simulink model "tqdtqr_rebuild_V3"  (R2021b)
settings: Solver=VariableStepAuto  StartTime=0.0  StopTime=10.0  RelTol=1e-3
undefined symbols (not defined in the file): ATQD_AfterTqMinGain_X_Deg, ATQD_APSCreepBaseTqD_X_kph, ATQD_APSCreepBaseTqD_Y_Deg, ATQD_APSCreepBaseTqR_X_kph, ATQD_APSCreepBaseTqR_Y_Deg, ATQD_APSCreepIterm_X_kph, ATQD_APSCreepIterm_Y_kph, ATQD_APSCreepPterm_X_kph, ATQD_APSCreepPterm_Y_kph, ATQD_APSDecReq_X_kph, ATQD_APSDecReq_Y_mps2, ATQD_APSDecReqCMD_X_kph, ATQD_APSDecReqTs_X_pct, ATQD_APSDecTimeGain_X_Deg, ATQD_APSDecTimeGain_Y_s, ATQD_APSReqLowSpd_X_Deg, ATQD_AutoHoldReleaseBPS_X_Deg, ATQD_AWDLoadTrqnsGain_X_kg, ATQD_AWDLoadTrqnsGain_Y_pct, ATQD_BOSEnBPSPosn_X_kph, ATQD_BOSMap_X_rpm, ATQD_BOSMap_Y_pct, ATQD_CreepBaseTqD_X_kph, ATQD_CreepBaseTqD_Y_Deg, ATQD_CreepBaseTqR_X_kph, ATQD_CreepBaseTqR_Y_Deg, ATQD_CreepBPSDisPosn_X_Deg, ATQD_CreepBPSDisPosnR_X_Deg, ATQD_CreepBPSEnPosn_X_Deg, ATQD_CreepBPSEnPosnR_X_Deg, ATQD_CreepDeltaTq_X_kph, ATQD_CreepIterm_X_kph, ATQD_CreepIterm_Y_kph, ATQD_CreepItermMaxLimit_X_pct, ATQD_CreepPreloadTime_X_kph, ATQD_CreepPreloadTq_X_kph, ATQD_CreepPreloadTq_Y_s, ATQD_CreepProtTq_X_Deg, ATQD_CreepPterm_X_kph, ATQD_CreepPterm_Y_kph, ATQD_CreepRrTqSpRat_X_rpm, ATQD_CreepRrTqSpRat_Y_Nm, ATQD_CreepTargetSpdD_X_pct, ATQD_CreepTargetSpdR_X_pct, ATQD_CreepUpLimitTq_X_rpm, ATQD_DecIneOPDHoldEnDelay_X_Deg, ATQD_DecIneOPDHoldEnDelay_Y_bar, ATQD_ECOTqMapD_X_rpm, ATQD_ECOTqMapD_Y_pct, ATQD_EMTqMapD_X_rpm, ATQD_EMTqMapD_Y_pct, ATQD_EOPDTqMapDCon_X_rpm, ATQD_EOPDTqMapDCon_Y_Deg, ATQD_EstInitVehWeight_X_c, ATQD_FAfterTqCMDGain_X_rpm, ATQD_FAfterTqCMDGain_Y_pct, ATQD_ForceLowSpd_X_Deg, ATQD_ForcePLimitSpd_X_Deg, ATQD_FrLossMAPLowV_X_rpm, ATQD_FrLossMAPLowV_Y_Nm ... (+949)
libraries: simulink x235, hcu_lib x208, tqr x63, tqd x6
(part 21 of 37)

== system tqdtqr_rebuild_V3/Input_Convert/Main function/Front//Rear zero point transfer/Negative Rate limit Determination ==
  VTQD_TqTargetShaftSpd_rpm : Inport
  VTQR_FEDUWhlTqReqSmoothDelay_Nm : Inport  Port=2
  VTQR_EVDriveMode_enum : Inport  Port=3
  Constant1 : Constant  Value=ENUM_DRIVEMODE_ECO
  Constant2 : Constant  Value=ENUM_DRIVEMODE_NRM
  Constant3 : Constant  Value=ENUM_DRIVEMODE_SPORT
  Constant7 : Constant  Value=ENUM_DRIVEMODE_ECO
  Constant8 : Constant  Value=ENUM_DRIVEMODE_NRM
  Constant9 : Constant  Value=ENUM_DRIVEMODE_SPORT
  Equal{1..3,5..6,8} (6 alike) : RelationalOperator  Operator===  OutDataTypeStr=boolean  RndMeth=Simplest
  If1 : If  NumInputs=3  IfExpression=u1~= 0  ElseIfExpressions=u2 ~= 0, u3 ~= 0  ShowElse=off
  If2 : If  NumInputs=3  IfExpression=u1~= 0  ElseIfExpressions=u2 ~= 0, u3 ~= 0  ShowElse=off
  Merge1 : Merge  Inputs=3
  Merge2 : Merge  Inputs=3
  Mux : Mux  Inputs=2
  VTQR_FrNegRateLimitDecE_Nm : Subsystem  TreatAsAtomicUnit=on
  VTQR_FrNegRateLimitDecN_Nm : Subsystem  TreatAsAtomicUnit=on
  VTQR_FrNegRateLimitDecS_Nm : Subsystem  TreatAsAtomicUnit=on
  VTQR_FrNegRateLimitIncE_Nm : Subsystem  TreatAsAtomicUnit=on
  VTQR_FrNegRateLimitIncN_Nm : Subsystem  TreatAsAtomicUnit=on
  VTQR_FrNegRateLimitIncS_Nm : Subsystem  TreatAsAtomicUnit=on
  VTQR_NegRateLimit_mux : Outport
  wires:
  VTQR_EVDriveMode_enum/1 -> [VTQR_EVDriveMode_enum]
  VTQR_FEDUWhlTqReqSmoothDelay_Nm/1 -> [VTQR_FEDUWhlTqReqSmoothDelay_Nm]
  VTQD_TqTargetShaftSpd_rpm/1 -> [VTQD_TqTargetShaftSpd_rpm]
  Mux/1 -> VTQR_NegRateLimit_mux/1  "VTQR_NegRateLimit_mux"
  Merge1/1 -> Mux/1  "VTQR_NegRateLimitInc_Nm"
  Constant7/1 -> Equal5/2
  Constant9/1 -> Equal8/2
  Constant8/1 -> Equal6/2
  [VTQR_EVDriveMode_enum] -> Equal5/1
  [VTQR_EVDriveMode_enum] -> Equal8/1
  [VTQR_EVDriveMode_enum] -> Equal6/1
  Equal6/1 -> If1/1
  Equal5/1 -> If1/2
  Equal8/1 -> If1/3
  [VTQD_TqTargetShaftSpd_rpm] -> VTQR_FrNegRateLimitIncN_Nm/1(VTQD_TqTargetShaftSpd_rpm)
  [VTQR_FEDUWhlTqReqSmoothDelay_Nm] -> VTQR_FrNegRateLimitIncN_Nm/2(VTQR_FEDUWhlTqReqSmoothDelay_Nm)
  If1/1 -> VTQR_FrNegRateLimitIncN_Nm/Action
  VTQR_FrNegRateLimitIncN_Nm/1(VTQR_FrNegRateLimitIncN_Nm) -> Merge1/1
  [VTQD_TqTargetShaftSpd_rpm] -> VTQR_FrNegRateLimitIncE_Nm/1(VTQD_TqTargetShaftSpd_rpm)
  [VTQR_FEDUWhlTqReqSmoothDelay_Nm] -> VTQR_FrNegRateLimitIncE_Nm/2(VTQR_FEDUWhlTqReqSmoothDelay_Nm)
  [VTQR_FEDUWhlTqReqSmoothDelay_Nm] -> VTQR_FrNegRateLimitIncS_Nm/2(VTQR_FEDUWhlTqReqSmoothDelay_Nm)
  [VTQD_TqTargetShaftSpd_rpm] -> VTQR_FrNegRateLimitIncS_Nm/1(VTQD_TqTargetShaftSpd_rpm)
  If1/3 -> VTQR_FrNegRateLimitIncS_Nm/Action
  If1/2 -> VTQR_FrNegRateLimitIncE_Nm/Action
  VTQR_FrNegRateLimitIncS_Nm/1(VTQR_FrNegRateLimitIncS_Nm) -> Merge1/3
  VTQR_FrNegRateLimitIncE_Nm/1(VTQR_FrNegRateLimitIncE_Nm) -> Merge1/2
  VTQR_FrNegRateLimitDecN_Nm/1(VTQR_FrNegRateLimitDecN_Nm) -> Merge2/1
  If2/3 -> VTQR_FrNegRateLimitDecS_Nm/Action
  Equal1/1 -> If2/2
  VTQR_FrNegRateLimitDecS_Nm/1(VTQR_FrNegRateLimitDecS_Nm) -> Merge2/3
  [VTQD_TqTargetShaftSpd_rpm] -> VTQR_FrNegRateLimitDecS_Nm/1(VTQD_TqTargetShaftSpd_rpm)
  [VTQR_FEDUWhlTqReqSmoothDelay_Nm] -> VTQR_FrNegRateLimitDecS_Nm/2(VTQR_FEDUWhlTqReqSmoothDelay_Nm)
  If2/1 -> VTQR_FrNegRateLimitDecN_Nm/Action
  [VTQR_FEDUWhlTqReqSmoothDelay_Nm] -> VTQR_FrNegRateLimitDecE_Nm/2(VTQR_FEDUWhlTqReqSmoothDelay_Nm)
  VTQR_FrNegRateLimitDecE_Nm/1(VTQR_FrNegRateLimitDecE_Nm) -> Merge2/2
  [VTQR_EVDriveMode_enum] -> Equal2/1
  [VTQR_EVDriveMode_enum] -> Equal3/1
  If2/2 -> VTQR_FrNegRateLimitDecE_Nm/Action
  Equal3/1 -> If2/3
  Constant3/1 -> Equal3/2
  Constant2/1 -> Equal2/2
  Equal2/1 -> If2/1
  [VTQR_EVDriveMode_enum] -> Equal1/1
  [VTQD_TqTargetShaftSpd_rpm] -> VTQR_FrNegRateLimitDecN_Nm/1(VTQD_TqTargetShaftSpd_rpm)
  [VTQR_FEDUWhlTqReqSmoothDelay_Nm] -> VTQR_FrNegRateLimitDecN_Nm/2(VTQR_FEDUWhlTqReqSmoothDelay_Nm)
  [VTQD_TqTargetShaftSpd_rpm] -> VTQR_FrNegRateLimitDecE_Nm/1(VTQD_TqTargetShaftSpd_rpm)
  Constant1/1 -> Equal1/2
  Merge2/1 -> Mux/2  "VTQR_NegRateLimitDec_Nm"

== system tqdtqr_rebuild_V3/Input_Convert/Main function/Front//Rear zero point transfer/Negative Rate limit Determination1 ==
  VTQD_TqTargetShaftSpd_rpm : Inport
  VTQR_REDUWhlTqReqSmoothDelay_Nm : Inport  Port=2
  VTQR_EVDriveMode_enum : Inport  Port=3
  Constant1 : Constant  Value=ENUM_DRIVEMODE_ECO
  Constant2 : Constant  Value=ENUM_DRIVEMODE_NRM
  Constant3 : Constant  Value=ENUM_DRIVEMODE_SPORT
  Constant7 : Constant  Value=ENUM_DRIVEMODE_ECO
  Constant8 : Constant  Value=ENUM_DRIVEMODE_NRM
  Constant9 : Constant  Value=ENUM_DRIVEMODE_SPORT
  Equal{1..3,5..6,8} (6 alike) : RelationalOperator  Operator===  OutDataTypeStr=boolean  RndMeth=Simplest
  If1 : If  NumInputs=3  IfExpression=u1~= 0  ElseIfExpressions=u2 ~= 0, u3 ~= 0  ShowElse=off
  If2 : If  NumInputs=3  IfExpression=u1~= 0  ElseIfExpressions=u2 ~= 0, u3 ~= 0  ShowElse=off
  Merge1 : Merge  Inputs=3
  Merge2 : Merge  Inputs=3
  Mux : Mux  Inputs=2
  VTQR_RrNegRateLimitDecE_Nm : Subsystem  TreatAsAtomicUnit=on
  VTQR_RrNegRateLimitDecN_Nm : Subsystem  TreatAsAtomicUnit=on
  VTQR_RrNegRateLimitDecS_Nm : Subsystem  TreatAsAtomicUnit=on
  VTQR_RrNegRateLimitIncE_Nm : Subsystem  TreatAsAtomicUnit=on
  VTQR_RrNegRateLimitIncN_Nm : Subsystem  TreatAsAtomicUnit=on
  VTQR_RrNegRateLimitIncS_Nm : Subsystem  TreatAsAtomicUnit=on
  VTQR_NegRateLimit_mux : Outport
  wires:
  Merge2/1 -> Mux/2  "VTQR_NegRateLimitDec_Nm"
  Constant1/1 -> Equal1/2
  [VTQD_TqTargetShaftSpd_rpm] -> VTQR_RrNegRateLimitDecE_Nm/1(VTQD_TqTargetShaftSpd_rpm)
  [VTQR_REDUWhlTqReqSmoothDelay_Nm] -> VTQR_RrNegRateLimitDecN_Nm/2(VTQR_REDUWhlTqReqSmoothDelay_Nm)
  [VTQD_TqTargetShaftSpd_rpm] -> VTQR_RrNegRateLimitDecN_Nm/1(VTQD_TqTargetShaftSpd_rpm)
  [VTQR_EVDriveMode_enum] -> Equal1/1
  Equal2/1 -> If2/1
  Constant2/1 -> Equal2/2
  Constant3/1 -> Equal3/2
  Equal3/1 -> If2/3
  If2/2 -> VTQR_RrNegRateLimitDecE_Nm/Action
  [VTQR_EVDriveMode_enum] -> Equal3/1
  [VTQR_EVDriveMode_enum] -> Equal2/1
  VTQR_RrNegRateLimitDecE_Nm/1(VTQR_RrNegRateLimitDecE_Nm) -> Merge2/2
  [VTQR_REDUWhlTqReqSmoothDelay_Nm] -> VTQR_RrNegRateLimitDecE_Nm/2(VTQR_REDUWhlTqReqSmoothDelay_Nm)
  If2/1 -> VTQR_RrNegRateLimitDecN_Nm/Action
  [VTQR_REDUWhlTqReqSmoothDelay_Nm] -> VTQR_RrNegRateLimitDecS_Nm/2(VTQR_REDUWhlTqReqSmoothDelay_Nm)
  [VTQD_TqTargetShaftSpd_rpm] -> VTQR_RrNegRateLimitDecS_Nm/1(VTQD_TqTargetShaftSpd_rpm)
  VTQR_RrNegRateLimitDecS_Nm/1(VTQR_RrNegRateLimitDecS_Nm) -> Merge2/3
  Equal1/1 -> If2/2
  If2/3 -> VTQR_RrNegRateLimitDecS_Nm/Action
  VTQR_RrNegRateLimitDecN_Nm/1(VTQR_RrNegRateLimitDecN_Nm) -> Merge2/1
  VTQR_RrNegRateLimitIncE_Nm/1(VTQR_RrNegRateLimitIncE_Nm) -> Merge1/2
  VTQR_RrNegRateLimitIncS_Nm/1(VTQR_RrNegRateLimitIncS_Nm) -> Merge1/3
  If1/2 -> VTQR_RrNegRateLimitIncE_Nm/Action
  If1/3 -> VTQR_RrNegRateLimitIncS_Nm/Action
  [VTQD_TqTargetShaftSpd_rpm] -> VTQR_RrNegRateLimitIncS_Nm/1(VTQD_TqTargetShaftSpd_rpm)
  [VTQR_REDUWhlTqReqSmoothDelay_Nm] -> VTQR_RrNegRateLimitIncS_Nm/2(VTQR_REDUWhlTqReqSmoothDelay_Nm)
  [VTQR_REDUWhlTqReqSmoothDelay_Nm] -> VTQR_RrNegRateLimitIncE_Nm/2(VTQR_REDUWhlTqReqSmoothDelay_Nm)
  [VTQD_TqTargetShaftSpd_rpm] -> VTQR_RrNegRateLimitIncE_Nm/1(VTQD_TqTargetShaftSpd_rpm)
  VTQR_RrNegRateLimitIncN_Nm/1(VTQR_RrNegRateLimitIncN_Nm) -> Merge1/1
  If1/1 -> VTQR_RrNegRateLimitIncN_Nm/Action
  [VTQR_REDUWhlTqReqSmoothDelay_Nm] -> VTQR_RrNegRateLimitIncN_Nm/2(VTQR_REDUWhlTqReqSmoothDelay_Nm)
  [VTQD_TqTargetShaftSpd_rpm] -> VTQR_RrNegRateLimitIncN_Nm/1(VTQD_TqTargetShaftSpd_rpm)
  Equal8/1 -> If1/3
  Equal5/1 -> If1/2
  Equal6/1 -> If1/1
  [VTQR_EVDriveMode_enum] -> Equal6/1
  [VTQR_EVDriveMode_enum] -> Equal8/1
  [VTQR_EVDriveMode_enum] -> Equal5/1
  Constant8/1 -> Equal6/2
  Constant9/1 -> Equal8/2
  Constant7/1 -> Equal5/2
  Merge1/1 -> Mux/1  "VTQR_NegRateLimitInc_Nm"
  Mux/1 -> VTQR_NegRateLimit_mux/1  "VTQR_NegRateLimit_mux"
  VTQD_TqTargetShaftSpd_rpm/1 -> [VTQD_TqTargetShaftSpd_rpm]
  VTQR_REDUWhlTqReqSmoothDelay_Nm/1 -> [VTQR_REDUWhlTqReqSmoothDelay_Nm]
  VTQR_EVDriveMode_enum/1 -> [VTQR_EVDriveMode_enum]

== system tqdtqr_rebuild_V3/Input_Convert/Main function/Front//Rear zero point transfer/Positive Rate limit Determination ==
  VTQD_TqTargetShaftSpd_rpm : Inport
  VTQR_FEDUWhlTqReqSmoothDelay_Nm : Inport  Port=2
  VTQR_EVDriveMode_enum : Inport  Port=3
  Constant1 : Constant  Value=ENUM_DRIVEMODE_ECO
  Constant2 : Constant  Value=ENUM_DRIVEMODE_NRM
  Constant3 : Constant  Value=ENUM_DRIVEMODE_SPORT
  Constant7 : Constant  Value=ENUM_DRIVEMODE_ECO
  Constant8 : Constant  Value=ENUM_DRIVEMODE_NRM
  Constant9 : Constant  Value=ENUM_DRIVEMODE_SPORT
  Equal{1..3,5..6,8} (6 alike) : RelationalOperator  Operator===  OutDataTypeStr=boolean  RndMeth=Simplest
  If1 : If  NumInputs=3  IfExpression=u1~= 0  ElseIfExpressions=u2 ~= 0, u3 ~= 0  ShowElse=off
  If2 : If  NumInputs=3  IfExpression=u1~= 0  ElseIfExpressions=u2 ~= 0, u3 ~= 0  ShowElse=off
  Merge1 : Merge  Inputs=3
  Merge2 : Merge  Inputs=3
  Mux : Mux  Inputs=2
  VTQR_FrPosRateLimitDecE_Nm : Subsystem  TreatAsAtomicUnit=on
  VTQR_FrPosRateLimitDecN_Nm : Subsystem  TreatAsAtomicUnit=on
  VTQR_FrPosRateLimitDecS_Nm : Subsystem  TreatAsAtomicUnit=on
  VTQR_FrPosRateLimitIncE_Nm : Subsystem  TreatAsAtomicUnit=on
  VTQR_FrPosRateLimitIncN_Nm : Subsystem  TreatAsAtomicUnit=on
  VTQR_FrPosRateLimitIncS_Nm : Subsystem  TreatAsAtomicUnit=on
  VTQR_PosRateLimit_mux : Outport
  wires:
  VTQR_EVDriveMode_enum/1 -> [VTQR_EVDriveMode_enum]
  VTQR_FEDUWhlTqReqSmoothDelay_Nm/1 -> [VTQR_FEDUWhlTqReqSmoothDelay_Nm]
  Merge2/1 -> Mux/2  "VTQR_PosRateLimitDec_Nm"
  Constant1/1 -> Equal1/2
  [VTQD_TqTargetShaftSpd_rpm] -> VTQR_FrPosRateLimitDecE_Nm/1(VTQD_TqTargetShaftSpd_rpm)
  [VTQR_FEDUWhlTqReqSmoothDelay_Nm] -> VTQR_FrPosRateLimitDecN_Nm/2(VTQR_FEDUWhlTqReqSmoothDelay_Nm)
  [VTQD_TqTargetShaftSpd_rpm] -> VTQR_FrPosRateLimitDecN_Nm/1(VTQD_TqTargetShaftSpd_rpm)
  [VTQR_EVDriveMode_enum] -> Equal1/1
  Equal2/1 -> If2/1
  Constant2/1 -> Equal2/2
  Constant3/1 -> Equal3/2
  Equal3/1 -> If2/3
  If2/2 -> VTQR_FrPosRateLimitDecE_Nm/Action
  [VTQR_EVDriveMode_enum] -> Equal3/1
  [VTQR_EVDriveMode_enum] -> Equal2/1
  VTQR_FrPosRateLimitDecE_Nm/1(VTQR_FrPosRateLimitDecE_Nm) -> Merge2/2
  [VTQR_FEDUWhlTqReqSmoothDelay_Nm] -> VTQR_FrPosRateLimitDecE_Nm/2(VTQR_FEDUWhlTqReqSmoothDelay_Nm)
  If2/1 -> VTQR_FrPosRateLimitDecN_Nm/Action
  [VTQR_FEDUWhlTqReqSmoothDelay_Nm] -> VTQR_FrPosRateLimitDecS_Nm/2(VTQR_FEDUWhlTqReqSmoothDelay_Nm)
  [VTQD_TqTargetShaftSpd_rpm] -> VTQR_FrPosRateLimitDecS_Nm/1(VTQD_TqTargetShaftSpd_rpm)
  VTQR_FrPosRateLimitDecS_Nm/1(VTQR_FrPosRateLimitDecS_Nm) -> Merge2/3
  Equal1/1 -> If2/2
  If2/3 -> VTQR_FrPosRateLimitDecS_Nm/Action
  VTQR_FrPosRateLimitDecN_Nm/1(VTQR_FrPosRateLimitDecN_Nm) -> Merge2/1
  VTQR_FrPosRateLimitIncE_Nm/1(VTQR_FrPosRateLimitIncE_Nm) -> Merge1/2
  VTQR_FrPosRateLimitIncS_Nm/1(VTQR_FrPosRateLimitIncS_Nm) -> Merge1/3
  If1/2 -> VTQR_FrPosRateLimitIncE_Nm/Action
  If1/3 -> VTQR_FrPosRateLimitIncS_Nm/Action
  [VTQD_TqTargetShaftSpd_rpm] -> VTQR_FrPosRateLimitIncS_Nm/1(VTQD_TqTargetShaftSpd_rpm)
  [VTQR_FEDUWhlTqReqSmoothDelay_Nm] -> VTQR_FrPosRateLimitIncS_Nm/2(VTQR_FEDUWhlTqReqSmoothDelay_Nm)
  [VTQR_FEDUWhlTqReqSmoothDelay_Nm] -> VTQR_FrPosRateLimitIncE_Nm/2(VTQR_FEDUWhlTqReqSmoothDelay_Nm)
  [VTQD_TqTargetShaftSpd_rpm] -> VTQR_FrPosRateLimitIncE_Nm/1(VTQD_TqTargetShaftSpd_rpm)
  VTQR_FrPosRateLimitIncN_Nm/1(VTQR_FrPosRateLimitIncN_Nm) -> Merge1/1
  If1/1 -> VTQR_FrPosRateLimitIncN_Nm/Action
  [VTQR_FEDUWhlTqReqSmoothDelay_Nm] -> VTQR_FrPosRateLimitIncN_Nm/2(VTQR_FEDUWhlTqReqSmoothDelay_Nm)
  [VTQD_TqTargetShaftSpd_rpm] -> VTQR_FrPosRateLimitIncN_Nm/1(VTQD_TqTargetShaftSpd_rpm)
  Equal8/1 -> If1/3
  Equal5/1 -> If1/2
  Equal6/1 -> If1/1
  [VTQR_EVDriveMode_enum] -> Equal6/1
  [VTQR_EVDriveMode_enum] -> Equal8/1
  [VTQR_EVDriveMode_enum] -> Equal5/1
  Constant8/1 -> Equal6/2
  Constant9/1 -> Equal8/2
  Constant7/1 -> Equal5/2
  Merge1/1 -> Mux/1  "VTQR_PosRateLimitInc_Nm"
  Mux/1 -> VTQR_PosRateLimit_mux/1  "VTQR_PosRateLimit_mux"
  VTQD_TqTargetShaftSpd_rpm/1 -> [VTQD_TqTargetShaftSpd_rpm]

== system tqdtqr_rebuild_V3/Input_Convert/Main function/Front//Rear zero point transfer/Positive Rate limit Determination1 ==
  VTQD_TqTargetShaftSpd_rpm : Inport
  VTQR_REDUWhlTqReqSmoothDelay_Nm : Inport  Port=2
  VTQR_EVDriveMode_enum : Inport  Port=3
  Constant1 : Constant  Value=ENUM_DRIVEMODE_ECO
  Constant2 : Constant  Value=ENUM_DRIVEMODE_NRM
  Constant3 : Constant  Value=ENUM_DRIVEMODE_SPORT
  Constant7 : Constant  Value=ENUM_DRIVEMODE_ECO
  Constant8 : Constant  Value=ENUM_DRIVEMODE_NRM
  Constant9 : Constant  Value=ENUM_DRIVEMODE_SPORT
  Equal{1..3,5..6,8} (6 alike) : RelationalOperator  Operator===  OutDataTypeStr=boolean  RndMeth=Simplest
  If1 : If  NumInputs=3  IfExpression=u1~= 0  ElseIfExpressions=u2 ~= 0, u3 ~= 0  ShowElse=off
  If2 : If  NumInputs=3  IfExpression=u1~= 0  ElseIfExpressions=u2 ~= 0, u3 ~= 0  ShowElse=off
  Merge1 : Merge  Inputs=3
  Merge2 : Merge  Inputs=3
  Mux : Mux  Inputs=2
  VTQR_RrPosRateLimitDecE_Nm : Subsystem  TreatAsAtomicUnit=on
  VTQR_RrPosRateLimitDecN_Nm : Subsystem  TreatAsAtomicUnit=on
  VTQR_RrPosRateLimitDecS_Nm : Subsystem  TreatAsAtomicUnit=on
  VTQR_RrPosRateLimitIncE_Nm : Subsystem  TreatAsAtomicUnit=on
  VTQR_RrPosRateLimitIncN_Nm : Subsystem  TreatAsAtomicUnit=on
  VTQR_RrPosRateLimitIncS_Nm : Subsystem  TreatAsAtomicUnit=on
  VTQR_PosRateLimit_mux : Outport
  wires:
  Mux/1 -> VTQR_PosRateLimit_mux/1  "VTQR_PosRateLimit_mux"
  Merge1/1 -> Mux/1  "VTQR_PosRateLimitInc_Nm"
  Constant7/1 -> Equal5/2
  Constant9/1 -> Equal8/2
  Constant8/1 -> Equal6/2
  [VTQR_EVDriveMode_enum] -> Equal5/1
  [VTQR_EVDriveMode_enum] -> Equal8/1
  [VTQR_EVDriveMode_enum] -> Equal6/1
  Equal6/1 -> If1/1
  Equal5/1 -> If1/2
  Equal8/1 -> If1/3
  [VTQD_TqTargetShaftSpd_rpm] -> VTQR_RrPosRateLimitIncN_Nm/1(VTQD_TqTargetShaftSpd_rpm)
  [VTQR_REDUWhlTqReqSmoothDelay_Nm] -> VTQR_RrPosRateLimitIncN_Nm/2(VTQR_REDUWhlTqReqSmoothDelay_Nm)
  If1/1 -> VTQR_RrPosRateLimitIncN_Nm/Action
  VTQR_RrPosRateLimitIncN_Nm/1(VTQR_RrPosRateLimitIncN_Nm) -> Merge1/1
  [VTQD_TqTargetShaftSpd_rpm] -> VTQR_RrPosRateLimitIncE_Nm/1(VTQD_TqTargetShaftSpd_rpm)
  [VTQR_REDUWhlTqReqSmoothDelay_Nm] -> VTQR_RrPosRateLimitIncE_Nm/2(VTQR_REDUWhlTqReqSmoothDelay_Nm)
  [VTQR_REDUWhlTqReqSmoothDelay_Nm] -> VTQR_RrPosRateLimitIncS_Nm/2(VTQR_REDUWhlTqReqSmoothDelay_Nm)
  [VTQD_TqTargetShaftSpd_rpm] -> VTQR_RrPosRateLimitIncS_Nm/1(VTQD_TqTargetShaftSpd_rpm)
  If1/3 -> VTQR_RrPosRateLimitIncS_Nm/Action
  If1/2 -> VTQR_RrPosRateLimitIncE_Nm/Action
  VTQR_RrPosRateLimitIncS_Nm/1(VTQR_RrPosRateLimitIncS_Nm) -> Merge1/3
  VTQR_RrPosRateLimitIncE_Nm/1(VTQR_RrPosRateLimitIncE_Nm) -> Merge1/2
  VTQR_RrPosRateLimitDecN_Nm/1(VTQR_RrPosRateLimitDecN_Nm) -> Merge2/1
  If2/3 -> VTQR_RrPosRateLimitDecS_Nm/Action
  Equal1/1 -> If2/2
  VTQR_RrPosRateLimitDecS_Nm/1(VTQR_RrPosRateLimitDecS_Nm) -> Merge2/3
  [VTQD_TqTargetShaftSpd_rpm] -> VTQR_RrPosRateLimitDecS_Nm/1(VTQD_TqTargetShaftSpd_rpm)
  [VTQR_REDUWhlTqReqSmoothDelay_Nm] -> VTQR_RrPosRateLimitDecS_Nm/2(VTQR_REDUWhlTqReqSmoothDelay_Nm)
  If2/1 -> VTQR_RrPosRateLimitDecN_Nm/Action
  [VTQR_REDUWhlTqReqSmoothDelay_Nm] -> VTQR_RrPosRateLimitDecE_Nm/2(VTQR_REDUWhlTqReqSmoothDelay_Nm)
  VTQR_RrPosRateLimitDecE_Nm/1(VTQR_RrPosRateLimitDecE_Nm) -> Merge2/2
  [VTQR_EVDriveMode_enum] -> Equal2/1
  [VTQR_EVDriveMode_enum] -> Equal3/1
  If2/2 -> VTQR_RrPosRateLimitDecE_Nm/Action
  Equal3/1 -> If2/3
  Constant3/1 -> Equal3/2
  Constant2/1 -> Equal2/2
  Equal2/1 -> If2/1
  [VTQR_EVDriveMode_enum] -> Equal1/1
  [VTQD_TqTargetShaftSpd_rpm] -> VTQR_RrPosRateLimitDecN_Nm/1(VTQD_TqTargetShaftSpd_rpm)
  [VTQR_REDUWhlTqReqSmoothDelay_Nm] -> VTQR_RrPosRateLimitDecN_Nm/2(VTQR_REDUWhlTqReqSmoothDelay_Nm)
  [VTQD_TqTargetShaftSpd_rpm] -> VTQR_RrPosRateLimitDecE_Nm/1(VTQD_TqTargetShaftSpd_rpm)
  Constant1/1 -> Equal1/2
  Merge2/1 -> Mux/2  "VTQR_PosRateLimitDec_Nm"
  VTQD_TqTargetShaftSpd_rpm/1 -> [VTQD_TqTargetShaftSpd_rpm]
  VTQR_REDUWhlTqReqSmoothDelay_Nm/1 -> [VTQR_REDUWhlTqReqSmoothDelay_Nm]
  VTQR_EVDriveMode_enum/1 -> [VTQR_EVDriveMode_enum]

== system tqdtqr_rebuild_V3/Input_Convert/Main function/Tq distribution function/AWD_Ratio ==
  VVMC_APSActive_flg : Inport
  VTQD_CreepPrLoadEnable_flg : Inport  Port=2
  VTQD_RrRatioWithRrSR_rat : Inport  Port=3
  VTQD_CreepEnable_flg : Inport  Port=4
  VTQD_OrigRrDriverRatio_rat : Inport  Port=5
  VTQD_CreepRrTqSpRat_rat : Inport  Port=6
  VTQD_RrTqSRRateTs_c : Inport  Port=7
  task_time_s : Inport  Port=8
  Action Port : ActionPort  ActionPortLabel=elseif(u2 ~= 0)
  AND : Logic  AllPortsSameDT=off  OutDataTypeStr=boolean
  AND2 : Logic  AllPortsSameDT=off  OutDataTypeStr=boolean
  Constant : Constant  Value=ONE_FLOAT
  Constant10 : Constant  Value=KTQD_AWDRrRatio_rat_ovrdflg  VectorParams1D=off  SampleTime=-1
  Constant11 : Constant  Value=KTQD_AWDRrRatio_rat_ovrdval  VectorParams1D=off  SampleTime=-1
  Constant12 : Constant  Value=KTQD_DrvSelPwrTrainSW_flg  VectorParams1D=off  SampleTime=-1
  Constant14 : Constant  Value=KTQD_CreepWhlRatioSW_flg
  Constant17 : Constant  Value=KTQD_AWDTqRatioSW_enum
  Constant18 : Constant  Value=KTQD_DriverSelPowerTrain_enum
  Constant19 : Constant  OutDataTypeStr=uint8
  Constant20 : Constant  Value=KTQD_AWDTqRatioSW_enum
  Constant21 : Constant  Value=2  OutDataTypeStr=uint8
  Constant3 : Constant  Value=ENUM_DRIVETRAIN_FWD  VectorParams1D=off  SampleTime=-1
  Constant4 : Constant  Value=ENUM_DRIVETRAIN_AWD  VectorParams1D=off  SampleTime=-1
  Constant6 : Constant  Value=KTQD_AWDFWDSelRRatio_rat  VectorParams1D=off  SampleTime=-1
  Constant7 : Constant  Value=KTQD_AWDRWDSelRRatio_rat  VectorParams1D=off  SampleTime=-1
  Constant8 : Constant  Value=KTQD_AWDFrRatio_rat_ovrdflg  VectorParams1D=off  SampleTime=-1
  Constant9 : Constant  Value=KTQD_AWDFrRatio_rat_ovrdval  VectorParams1D=off  SampleTime=-1
  Equal1 : RelationalOperator  Operator=~=  OutDataTypeStr=boolean  RndMeth=Simplest
  Equal3 : RelationalOperator  Operator===  OutDataTypeStr=boolean  RndMeth=Simplest
  Equal6 : RelationalOperator  Operator===  OutDataTypeStr=boolean  RndMeth=Simplest
  Equal7 : RelationalOperator  Operator===  OutDataTypeStr=boolean  RndMeth=Simplest
  FirstOrderFilter : hcu_lib/Basic_Blocks/FirstOrderFilter
  LiuzgSwitch2 : Switch  Criteria=u2 ~= 0
      settings: AttributesFormatString=<%<Criteria>>
  LiuzgSwitch4 : Switch  Criteria=u2 ~= 0
      settings: AttributesFormatString=<%<Criteria>>
  LiuzgSwitch5 : Switch  Criteria=u2 ~= 0
      settings: AttributesFormatString=<%<Criteria>>
  OR : Logic  Operator=OR  AllPortsSameDT=off  OutDataTypeStr=boolean
  OR1 : Logic  AllPortsSameDT=off  OutDataTypeStr=boolean
  OR3 : Logic  Operator=OR  AllPortsSameDT=off  OutDataTypeStr=boolean
  Saturation : Saturate  UpperLimit=KTQD_RrEDUTqDistrictMax_gain  LowerLimit=KTQD_RrEDUTqDistrictMin_gain
      settings: AttributesFormatString=|
      | <%<UpperLimit>>
      | <%<LowerLimit>>
  Subtract : Sum  Inputs=+-
  Switch : Switch  Criteria=u2 > Threshold
  Switch1 : Switch  Criteria=u2 > Threshold
  Switch3 : Switch  Criteria=u2 > Threshold
  VTQD_FrRatio_AWD : Outport
  VTQD_RrRatio_AWD : Outport  Port=2
  wires:
  [VTQD_RrTqSRRateTs_c] -> FirstOrderFilter/3
  [task_time_s] -> FirstOrderFilter/2
  FirstOrderFilter/1 -> LiuzgSwitch4/3
  LiuzgSwitch2/1 -> FirstOrderFilter/1
  task_time_s/1 -> [task_time_s]
  VTQD_RrTqSRRateTs_c/1 -> [VTQD_RrTqSRRateTs_c]
  [VTQD_CreepRrTqSpRat_rat] -> LiuzgSwitch2/1
  VTQD_CreepRrTqSpRat_rat/1 -> [VTQD_CreepRrTqSpRat_rat]
  VTQD_OrigRrDriverRatio_rat/1 -> [VTQD_OrigRrDriverRatio_rat]
  OR3/1 -> Switch3/2
  Equal7/1 -> OR3/2
  Constant20/1 -> Equal7/1
  Constant21/1 -> Equal7/2
  AND2/1 -> OR3/1
  [VTQD_CreepEnable_flg] -> AND2/2
  Equal6/1 -> AND2/1
  Constant19/1 -> Equal6/2
  Constant17/1 -> Equal6/1
  [VTQD_RrRatioWithRrSR_rat] -> Switch3/1
  [VTQD_OrigRrDriverRatio_rat] -> Switch3/3
  Switch3/1 -> LiuzgSwitch2/3  "VTQD_FitRrDriverRatio_rat"
  Constant6/1 -> LiuzgSwitch5/1
  Constant7/1 -> LiuzgSwitch5/3
  VTQD_RrRatioWithRrSR_rat/1 -> [VTQD_RrRatioWithRrSR_rat]
  VTQD_CreepEnable_flg/1 -> [VTQD_CreepEnable_flg]
  Constant14/1 -> OR1/2
  OR1/1 -> LiuzgSwitch2/2
  AND/1 -> LiuzgSwitch4/2
  Equal1/1 -> AND/1
  Constant12/1 -> AND/2
  Constant10/1 -> Switch1/2
  Constant11/1 -> Switch1/1
  Constant9/1 -> Switch/1
  Constant8/1 -> Switch/2
  Switch1/1 -> VTQD_RrRatio_AWD/1
  Switch/1 -> VTQD_FrRatio_AWD/1
  Subtract/1 -> Switch/3
  Constant18/1 -> [VINP_DriverSelPowerTrain_enum]  "VINP_DriverSelPowerTrain_enum"
  LiuzgSwitch4/1 -> Saturation/1
  Equal3/1 -> LiuzgSwitch5/2
  [VINP_DriverSelPowerTrain_enum] -> Equal3/1
  Constant3/1 -> Equal3/2
  LiuzgSwitch5/1 -> LiuzgSwitch4/1
  Constant4/1 -> Equal1/2
  [VINP_DriverSelPowerTrain_enum] -> Equal1/1
  VTQD_CreepPrLoadEnable_flg/1 -> [VTQD_CreepPrLoadEnable_flg]
  VVMC_APSActive_flg/1 -> [VVMC_APSActive_flg]
  [VVMC_APSActive_flg] -> OR/1
  [VTQD_CreepPrLoadEnable_flg] -> OR/2
  OR/1 -> OR1/1
  Saturation/1 -> Subtract/2, Switch1/3
  Constant/1 -> Subtract/1

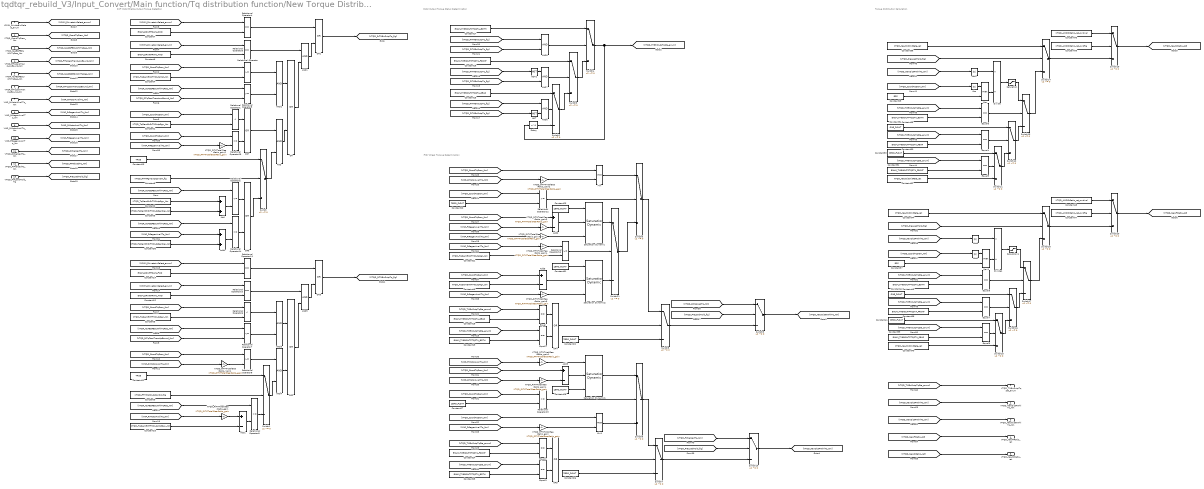
== system tqdtqr_rebuild_V3/Input_Convert/Main function/Tq distribution function/New Torque Distribution ==
  note: Rr/Fr Motor Enable Output Torque Detection
  note: Motor Output Torque Status Determination
  note: Fr/Rr Wheel Torqrue Determination
  note: Torque Distribution Calculation
  VPMM_DrivetrainSelect_enum : Inport
  VTQD_CoordTqDem_Nm : Inport  Port=2
  VTQR_NoABSFEDUWhlTqReq_Nm : Inport  Port=3
  VTQR_FrTqZeroTransLowBound_Nm : Inport  Port=4
  VTQR_NoABSREDUWhlTqReq_Nm : Inport  Port=5
  VTQR_RrTqZeroTransUpBound_Nm : Inport  Port=6
  VINP_RrMotorAvailTq_Nm : Inport  Port=7
  VINP_RrRegenAvailTq_Nm : Inport  Port=8
  VINP_FrMotorAvailTq_Nm : Inport  Port=9
  VINP_FrRegenAvailTq_Nm : Inport  Port=10
  VTQD_RrPreloadTq_Nm : Inport  Port=11
  VTQD_FrPreloadTq_Nm : Inport  Port=12
  VTQD_PreLoadHold_flg : Inport  Port=13
  AND{,1..8} (9 alike) : Logic  AllPortsSameDT=off  OutDataTypeStr=boolean
  Abs{,1..3} (4 alike) : Abs
  Add : Sum
  Add{1..3,5} (4 alike) : Sum  Inputs=+-
  Add4 : Sum
  Constant{1..2,21,49} (4 alike) : Constant  Value=KTQD_TqDemEnRrTMOutpRgn_Nm
  Constant10 : Constant  Value=KTQD_TqDemEnFrTMOutpMotDev_Nm
  Constant11 : Constant  Value=TRUE
  Constant12 : Constant  Value=ENUM_DRIVETRAIN_AWD
  Constant13 : Constant  Value=TRUE
  Constant14 : Constant  Value=ENUM_DRIVETRAIN_FWD
  Constant{15,18,30,39} (4 alike) : Constant  Value=ENUM_TMENOUTPTQSTA_REAR
  Constant{16,24,31,38} (4 alike) : Constant  Value=ENUM_TMENOUTPTQSTA_FRONT
  Constant{17,19,25,35,43} (5 alike) : Constant  Value=ENUM_TMENOUTPTQSTA_BOTH
  Constant{20,22..23,26..28,33,41,51} (9 alike) : Constant  Value=ZERO_FLOAT
  Constant29 : Constant  Value=EPS
  Constant3 : Constant  Value=KTQD_TqDemEnRrTMOutpRgnDev_Nm
  Constant{32,36,40,44} (4 alike) : Constant  Value=KTQD_NewDistInitRate_rat
  Constant34 : Constant  Value=ONE_FLOAT
  Constant37 : Constant  Value=EPS
  Constant4 : Constant  Value=KTQD_TqDemEnRrTMOutpMot_Nm
  Constant42 : Constant  Value=ONE_FLOAT
  Constant45 : Constant  Value=KTQD_AWDRrRatio_rat_ovrdflg
  Constant46 : Constant  Value=KTQD_AWDRrRatio_rat_ovrdval
  Constant47 : Constant  Value=KTQD_AWDRrRatio_rat_ovrdflg
  Constant48 : Constant  Value=KTQD_AWDRrRatio_rat_ovrdval
  Constant5 : Constant  Value=KTQD_TqDemEnFrTMOutpRgn_Nm
  Constant50 : Constant  Value=KTQD_TqDemEnRrTMOutpRgnDev_Nm
  Constant6 : Constant  Value=ENUM_DRIVETRAIN_AWD
  Constant7 : Constant  Value=ENUM_DRIVETRAIN_RWD
  Constant8 : Constant  Value=KTQD_RrTMRgnOutpConSW_flg
  Constant9 : Constant  Value=KTQD_FrTMMotOutpConSW_flg
  Delay : Delay  DelayLength=1  InitialCondition=uint8(0)
      settings: AttributesFormatString=%<InitialCondition>
  Divide : Product  Inputs=*/
  Divide1 : Product  Inputs=*/
  Equal{,1..9} (10 alike) : RelationalOperator  Operator===  OutDataTypeStr=boolean  RndMeth=Simplest
  KTQD_FrTMTotalGearRatio_gain{,1..4} (5 alike) : Gain  Gain=KTQD_FrTMTotalGearRatio_gain
  KTQD_RrTMTotalGearRatio_gain{,1..5} (6 alike) : Gain  Gain=KTQD_RrTMTotalGearRatio_gain
  Max : MinMax  Function=max  Inputs=2
  Max1 : MinMax  Function=max  Inputs=2
  Min : MinMax  Inputs=2
  Min1 : MinMax  Function=max  Inputs=2
  NOT : Logic  Operator=NOT  AllPortsSameDT=off  OutDataTypeStr=boolean
  NOT2 : Logic  Operator=NOT  AllPortsSameDT=off  OutDataTypeStr=boolean
  OR{,1..7} (8 alike) : Logic  Operator=OR  AllPortsSameDT=off  OutDataTypeStr=boolean
  Relational Operator{,5,8..9,12..13,16} (7 alike) : RelationalOperator  OutDataTypeStr=boolean  RndMeth=Simplest
  Relational Operator1 : RelationalOperator  Operator=<  OutDataTypeStr=boolean  RndMeth=Simplest
  Relational Operator{3..4,10..11} (4 alike) : RelationalOperator  Operator===  OutDataTypeStr=boolean  RndMeth=Simplest
  Relational Operator{2,7,14..15} (4 alike) : RelationalOperator  Operator=<=  OutDataTypeStr=boolean  RndMeth=Simplest
  Relational Operator6 : RelationalOperator  Operator=<  OutDataTypeStr=boolean  RndMeth=Simplest
  Saturation : Saturate  UpperLimit=single(1)  LowerLimit=single(0)
      settings: AttributesFormatString=|
      | UpperLimit:%<UpperLimit>
      | LowerLimi:%<LowerLimit>
  Saturation Dynamic : simulink/Discontinuities/Saturation Dynamic  OutMin=[]  OutMax=[]  OutDataTypeStr=Inherit: Same as second input  OutDataType=fixdt(1, 16)  OutScaling=2^-10  DoSatur=off
  Saturation Dynamic1 : simulink/Discontinuities/Saturation Dynamic  OutMin=[]  OutMax=[]  OutDataTypeStr=Inherit: Same as second input  OutDataType=fixdt(1, 16)  OutScaling=2^-10  DoSatur=off
  Saturation Dynamic2 : simulink/Discontinuities/Saturation Dynamic  OutMin=[]  OutMax=[]  OutDataTypeStr=Inherit: Same as second input  OutDataType=fixdt(1, 16)  OutScaling=2^-10  DoSatur=off
  Saturation1 : Saturate  UpperLimit=single(1)  LowerLimit=single(0)
      settings: AttributesFormatString=|
      | UpperLimit:%<UpperLimit>
      | LowerLimi:%<LowerLimit>
  Switch{,1..21} (22 alike) : Switch  Criteria=u2 ~= 0
      settings: AttributesFormatString=%<Criteria>
  VTQD_TMEnOutpTqSta_enum : Outport
  VTQD_NewDistFrWhlTq_Nm : Outport  Port=2
  VTQD_NewDistRrWhlTq_Nm : Outport  Port=3
  VTQD_NewFrRatio_rat : Outport  Port=4
  VTQD_NewRrRatio_rat : Outport  Port=5
  wires:
  VTQD_CoordTqDem_Nm/1 -> [VTQD_CoordTqDem_Nm]
  [VTQD_TMEnOutpTqSta_enum] -> VTQD_TMEnOutpTqSta_enum/1
  Constant21/1 -> Relational Operator16/2
  [VTQD_NewDistRrWhlTq_Nm] -> VTQD_NewDistRrWhlTq_Nm/1
  Relational Operator1/1 -> OR7/1
  VTQD_RrPreloadTq_Nm/1 -> [VTQD_RrPreloadTq_Nm]
  [VTQD_NewDistFrWhlTq_Nm] -> VTQD_NewDistFrWhlTq_Nm/1
  VTQR_NoABSFEDUWhlTqReq_Nm/1 -> [VTQR_NoABSFEDUWhlTqReq_Nm]
  Switch19/1 -> [VTQD_NewRrRatio_rat]  "VTQD_NewRrRatio_rat"
  Relational Operator14/1 -> OR6/2
  OR7/1 -> AND/1
  Add4/1 -> Relational Operator14/2
  Constant50/1 -> Add4/2
  VINP_RrRegenAvailTq_Nm/1 -> [VINP_RrRegenAvailTq_Nm]
  VTQD_PreLoadHold_flg/1 -> [VTQD_PreLoadHold_flg]
  Switch21/1 -> Switch6/3
  Saturation Dynamic/1 -> Switch21/1
  KTQD_FrTMTotalGearRatio_gain3/1 -> Add2/2
  [VTQD_CoordTqDem_Nm] -> Relational Operator15/1
  Switch13/1 -> Switch14/3
  Constant47/1 -> Switch20/2
  Constant49/1 -> Add5/2
  [VINP_RrRegenAvailTq_Nm] -> KTQD_RrTMTotalGearRatio_gain5/1
  [VTQD_PreLoadHold_flg] -> Switch14/2
  Equal6/1 -> Switch13/2
  Constant15/1 -> Switch2/1
  [VTQD_NewRrRatio_rat] -> VTQD_NewRrRatio_rat/1
  Add5/1 -> Saturation Dynamic2/2
  Saturation/1 -> Switch13/1
  [VINP_FrRegenAvailTq_Nm] -> KTQD_FrTMTotalGearRatio_gain/1
  [VINP_FrRegenAvailTq_Nm] -> KTQD_FrTMTotalGearRatio_gain3/1
  Constant24/1 -> Equal2/2
  Constant33/1 -> Switch11/1
  Constant23/1 -> Saturation Dynamic/1
  Constant30/1 -> Equal4/2
  [VTQD_NewDistRrWhlTq_Nm] -> Abs1/1
  Saturation Dynamic1/1 -> Switch8/1
  Constant22/1 -> Switch5/3
  KTQD_RrTMTotalGearRatio_gain1/1 -> Relational Operator8/2
  [VINP_FrRegenAvailTq_Nm] -> Add4/1
  Relational Operator10/1 -> AND5/1
  Constant32/1 -> Switch11/3
  Abs1/1 -> Divide/1
  Switch1/1 -> AND4/2
  Divide/1 -> Saturation/1
  Constant19/1 -> Equal1/2
  [VTQD_FrTMEnOutpTq_flg] -> AND7/2
  KTQD_FrTMTotalGearRatio_gain1/1 -> Saturation Dynamic1/1
  Constant29/1 -> Max/2
  KTQD_RrTMTotalGearRatio_gain3/1 -> Saturation Dynamic/3
  Max/1 -> Divide/2
  Constant27/1 -> Relational Operator13/2
  [VTQD_RrPreloadTq_Nm] -> Switch9/1
  [VTQD_CoordTqDem_Nm] -> Abs/1
  Constant46/1 -> Switch19/1
  Constant16/1 -> Switch3/1
  Constant5/1 -> Relational Operator6/2
  KTQD_FrTMTotalGearRatio_gain2/1 -> Relational Operator15/2
  [VINP_RrRegenAvailTq_Nm] -> KTQD_RrTMTotalGearRatio_gain3/1
  Switch8/1 -> Switch7/1
  Add3/1 -> Saturation Dynamic1/2
  [VPMM_DrivetrainSelect_enum] -> Relational Operator3/1
  Switch5/1 -> Switch9/3
  Switch7/1 -> Switch10/3
  Switch9/1 -> [VTQD_NewDistRrWhlTq_Nm]  "VTQD_NewDistRrWhlTq_Nm"
  Relational Operator13/1 -> Switch8/2
  [VTQR_NoABSFEDUWhlTqReq_Nm] -> Relational Operator14/1
  KTQD_FrTMTotalGearRatio_gain/1 -> Min1/2
  [VINP_FrMotorAvailTq_Nm] -> KTQD_FrTMTotalGearRatio_gain1/1
  [VTQD_CoordTqDem_Nm] -> Relational Operator8/1
  KTQD_RrTMTotalGearRatio_gain4/1 -> Add3/2
  Constant26/1 -> Switch7/3
  Min1/1 -> Switch8/3
  KTQD_FrTMTotalGearRatio_gain4/1 -> Relational Operator16/1
  Relational Operator4/1 -> OR1/1
  VTQR_FrTqZeroTransLowBound_Nm/1 -> [VTQR_FrTqZeroTransLowBound_Nm]
  VINP_FrMotorAvailTq_Nm/1 -> [VINP_FrMotorAvailTq_Nm]
  [VINP_RrMotorAvailTq_Nm] -> KTQD_RrTMTotalGearRatio_gain4/1
  Equal2/1 -> OR5/1
  Constant3/1 -> Add/2
  [VPMM_DrivetrainSelect_enum] -> Relational Operator11/1
  Min/1 -> Switch6/1
  Switch4/1 -> [VTQD_TMEnOutpTqSta_enum], Delay/1  "VTQD_TMEnOutpTqSta_enum"
  Constant35/1 -> Equal6/2
  Constant51/1 -> Saturation Dynamic2/1
  Switch6/1 -> Switch5/1
  KTQD_RrTMTotalGearRatio_gain2/1 -> Min/2
  [VTQD_CoordTqDem_Nm] -> Min/1
  [VTQD_TMEnOutpTqSta_enum] -> Equal6/1
  Relational Operator12/1 -> Switch6/2
  KTQD_RrTMTotalGearRatio_gain/1 -> Add1/1
  Constant25/1 -> Equal3/2
  Add2/1 -> Saturation Dynamic/2
  [VTQD_CoordTqDem_Nm] -> Relational Operator12/1
  [VINP_RrMotorAvailTq_Nm] -> KTQD_RrTMTotalGearRatio_gain2/1
  AND8/1 -> Switch4/2
  [VTQD_TMEnOutpTqSta_enum] -> Equal1/1
  OR4/1 -> Switch5/2
  Relational Operator11/1 -> OR3/1
  Constant20/1 -> Relational Operator12/2
  Switch3/1 -> Switch4/3
  Constant36/1 -> Switch14/1
  [VTQD_CoordTqDem_Nm] -> Relational Operator6/1
  [VTQD_FrTMEnOutpTq_flg] -> NOT/1
  OR5/1 -> Switch7/2
  Add1/1 -> Relational Operator9/2
  Constant9/1 -> Switch1/2
  [VTQD_CoordTqDem_Nm] -> Add2/1
  AND7/1 -> Switch3/2
  Constant18/1 -> Equal/2
  [VTQD_TMEnOutpTqSta_enum] -> Equal3/1
  Relational Operator2/1 -> OR6/1
  AND2/1 -> OR/1
  OR/1 -> AND1/2
  [VTQD_TMEnOutpTqSta_enum] -> Equal/1
  Equal5/1 -> Switch11/2
  [VTQD_RrTMEnOutpTq_flg] -> AND8/1
  [VTQD_RrTMEnOutpTq_flg] -> AND6/1
  VTQR_RrTqZeroTransUpBound_Nm/1 -> [VTQR_RrTqZeroTransUpBound_Nm]
  Constant17/1 -> Switch4/1
  NOT2/1 -> AND7/1
  Relational Operator15/1 -> OR7/2
  [VTQD_RrTMEnOutpTq_flg] -> NOT2/1
  Switch2/1 -> Switch3/3
  Constant11/1 -> Switch1/1
  [VTQD_TMEnOutpTqSta_enum] -> Equal2/1
  Relational Operator9/1 -> Switch1/3
  [VINP_RrMotorAvailTq_Nm] -> KTQD_RrTMTotalGearRatio_gain/1
  Relational Operator8/1 -> AND4/1
  AND5/1 -> OR3/2
  [VTQD_FrTMEnOutpTq_flg] -> AND8/2
  [VTQR_NoABSREDUWhlTqReq_Nm] -> Relational Operator9/1
  OR1/1 -> [VTQD_RrTMEnOutpTq_flg]  "VTQD_RrTMEnOutpTq_flg"
  [VTQR_NoABSREDUWhlTqReq_Nm] -> Relational Operator7/1
  [VPMM_DrivetrainSelect_enum] -> Relational Operator4/1
  AND/1 -> OR/2
  Relational Operator/1 -> AND2/1
  [VTQR_FrTqZeroTransLowBound_Nm] -> Relational Operator5/2
  Constant7/1 -> Relational Operator4/2
  AND1/1 -> OR1/2
  Equal/1 -> OR4/1
  Equal4/1 -> Switch12/2
  [VTQR_NoABSFEDUWhlTqReq_Nm] -> Relational Operator5/1
  [VPMM_DrivetrainSelect_enum] -> Relational Operator10/1
  [VTQD_TMEnOutpTqSta_enum] -> Equal4/1
  Constant45/1 -> Switch19/2
  Relational Operator7/1 -> AND3/2
  Delay/1 -> Switch2/3
  Add/1 -> Relational Operator2/2
  Switch14/1 -> Switch19/3  "VTQD_InitNewRrRatio_rat"
  VTQR_NoABSREDUWhlTqReq_Nm/1 -> [VTQR_NoABSREDUWhlTqReq_Nm]
  [VTQD_CoordTqDem_Nm] -> Relational Operator13/1
  Switch20/1 -> [VTQD_NewFrRatio_rat]  "VTQD_NewFrRatio_rat"
  Constant37/1 -> Max1/2
  Relational Operator5/1 -> AND2/2
  Constant6/1 -> Relational Operator3/2
  [VTQD_CoordTqDem_Nm] -> Abs2/1
  [VTQD_NewDistFrWhlTq_Nm] -> Abs3/1
  Constant13/1 -> Switch/1
  AND6/1 -> Switch2/2
  [VTQD_TMEnOutpTqSta_enum] -> Equal7/1
  Switch12/1 -> Switch13/3
  Switch/1 -> AND/2
  [VTQD_CoordTqDem_Nm] -> Relational Operator/1
  [VTQD_PreLoadHold_flg] -> Switch9/2
  [VINP_FrRegenAvailTq_Nm] -> KTQD_FrTMTotalGearRatio_gain2/1
  [VTQD_TMEnOutpTqSta_enum] -> Equal8/1
  Switch18/1 -> Switch20/3  "VTQD_InitNewFrRatio_rat"
  Divide1/1 -> Saturation1/1
  [VTQR_RrTqZeroTransUpBound_Nm] -> Relational Operator7/2
  [VTQD_CoordTqDem_Nm] -> Min1/1
  Abs3/1 -> Divide1/1
  [VTQD_TMEnOutpTqSta_enum] -> Equal5/1
  [VINP_FrRegenAvailTq_Nm] -> KTQD_FrTMTotalGearRatio_gain4/1
  Equal7/1 -> Switch16/2
  Max1/1 -> Divide1/2
  [VINP_RrMotorAvailTq_Nm] -> KTQD_RrTMTotalGearRatio_gain1/1
  Abs2/1 -> Max1/1
  Relational Operator3/1 -> AND1/1
  VINP_RrMotorAvailTq_Nm/1 -> [VINP_RrMotorAvailTq_Nm]
  Constant28/1 -> Saturation Dynamic1/3
  VINP_FrRegenAvailTq_Nm/1 -> [VINP_FrRegenAvailTq_Nm]
  [VTQD_TMEnOutpTqSta_enum] -> Equal9/1
  Switch15/1 -> Switch16/3
  KTQD_RrTMTotalGearRatio_gain5/1 -> Saturation Dynamic2/3
  VPMM_DrivetrainSelect_enum/1 -> [VPMM_DrivetrainSelect_enum]
  Switch16/1 -> Switch17/3
  [VTQD_CoordTqDem_Nm] -> Relational Operator1/1
  Constant43/1 -> Equal9/2
  OR3/1 -> [VTQD_FrTMEnOutpTq_flg]  "VTQD_FrTMEnOutpTq_flg"
  Constant2/1 -> Add/1
  [VTQR_NoABSFEDUWhlTqReq_Nm] -> Relational Operator2/1
  Switch11/1 -> Switch12/3
  Saturation1/1 -> Switch17/1
  OR6/1 -> Switch/3
  OR2/1 -> AND5/2
  Equal1/1 -> OR4/2
  Constant39/1 -> Equal8/2
  Constant48/1 -> Switch20/1
  Constant44/1 -> Switch18/1
  AND4/1 -> OR2/2
  Constant4/1 -> Relational Operator/2
  Constant31/1 -> Equal5/2
  [VTQD_NewFrRatio_rat] -> VTQD_NewFrRatio_rat/1
  [VTQD_PreLoadHold_flg] -> Switch18/2
  Constant40/1 -> Switch15/3
  Constant1/1 -> Relational Operator1/2
  Constant8/1 -> Switch/2
  [VTQD_FrPreloadTq_Nm] -> Switch10/1
  Relational Operator6/1 -> AND3/1
  Equal3/1 -> OR5/2
  Equal8/1 -> Switch15/2
  Switch10/1 -> [VTQD_NewDistFrWhlTq_Nm]  "VTQD_NewDistFrWhlTq_Nm"
  AND3/1 -> OR2/1
  Constant34/1 -> Switch12/1
  Switch17/1 -> Switch18/3
  Abs/1 -> Max/1
  Constant10/1 -> Add1/2
  Constant38/1 -> Equal7/2
  Constant41/1 -> Switch15/1
  Constant12/1 -> Relational Operator10/2
  Relational Operator16/1 -> Switch21/2
  Constant42/1 -> Switch16/1
  VTQD_FrPreloadTq_Nm/1 -> [VTQD_FrPreloadTq_Nm]
  NOT/1 -> AND6/2
  Constant14/1 -> Relational Operator11/2
  [VTQD_PreLoadHold_flg] -> Switch10/2
  Equal9/1 -> Switch17/2
  [VTQD_CoordTqDem_Nm] -> Add3/1
  Saturation Dynamic2/1 -> Switch21/3
  [VTQD_CoordTqDem_Nm] -> Add5/1

== system tqdtqr_rebuild_V3/Input_Convert/Signal function/OPD Hold/Deceleration Calculation ==
  VTQD_VehActSpd_kph : Inport
  VVMC_LongAcc_Gps : Inport  Port=2
  VTQD_APSReqTimer_s : Inport  Port=3
  VVMC_EstSlope_Deg : Inport  Port=4
  VTQD_APSDecReqA_flg : Inport  Port=5
  VTQD_AutiHoldRelease_flg : Inport  Port=6
  task_time_s : Inport  Port=7
  VTQD_ActAPSPosn_pct : Inport  Port=8
  VTQD_LowIdleAccPedal_flg : Inport  Port=9
  VTQD_OPDHoldForceEn_flg : Inport  Port=10
  AND1 : Logic  Inputs=3  AllPortsSameDT=off  OutDataTypeStr=boolean
  AND4 : Logic  Inputs=3  AllPortsSameDT=off  OutDataTypeStr=boolean
  Add : Sum  Inputs=+-
  Constant1 : Constant  Value=KTQD_APSDecReqMaxTime_s
  Constant13 : Constant  Value=ZERO_FLOAT
  Constant19 : Constant  Value=KTQD_OPDHoldBrkSW_flg
  Constant2 : Constant  Value=KTQD_OPDHoldBrkSW_flg
  Constant21 : Constant  Value=KTQD_OPDHoldDevUpLim_mps2
  Constant22 : Constant  Value=KTQD_OPDHoldDevLowLim_mps2
  Constant43 : Constant  Value=KTQD_APSDecReqMaxSW_flg
  Constant8 : Constant  Value=KVMC_GravityValue_mps2
  Delay : Delay  DelayLength=1
  FirstOrderFilter1 : tqr/TQR/Determine Torque Request/TorqueArbitrament/TorqueSmooth/FirstOrderFilter
  MTQD_APSDecReg_Z_mps2 : Lookup_n-D  BreakpointsForDimension1=ATQD_APSDecReq_Y_mps2  BreakpointsForDimension2=ATQD_APSDecReq_X_kph  Table=MTQD_APSDecReq_Z_mps2  InternalRulePriority=Speed  RndMeth=Simplest  InputSameDT=on
      settings: InputPortMap=u0,u1
  MTQD_APSDecReqCMD_Y_mps2 : Lookup_n-D  NumberOfTableDimensions=1  BreakpointsForDimension1=ATQD_APSDecReqCMD_X_kph  Table=MTQD_APSDecReqCMD_Y_mps2  InternalRulePriority=Speed  RndMeth=Simplest  InputSameDT=on
  MTQD_APSDecReqTs_Y_c : Lookup_n-D  NumberOfTableDimensions=1  BreakpointsForDimension1=ATQD_APSDecReqTs_X_pct  Table=MTQD_APSDecReqTs_Y_c  InternalRulePriority=Speed  RndMeth=Simplest  InputSameDT=on
  MTQD_APSDecTimeGain_Z_c : Lookup_n-D  BreakpointsForDimension1=ATQD_APSDecTimeGain_Y_s  BreakpointsForDimension2=ATQD_APSDecTimeGain_X_Deg  Table=MTQD_APSDecTimeGain_Z_c  InternalRulePriority=Speed  RndMeth=Simplest  InputSameDT=on
      settings: InputPortMap=u0,u1
  MTQD_ForceAPSDecReq_Z_mps2 : Lookup_n-D  BreakpointsForDimension1=ATQD_APSDecReq_Y_mps2  BreakpointsForDimension2=ATQD_APSDecReq_X_kph  Table=MTQD_ForceAPSDecReq_Z_mps2  InternalRulePriority=Speed  RndMeth=Simplest  InputSameDT=on
      settings: InputPortMap=u0,u1
  MTQD_ForceAPSDecTimeGain_Z_c : Lookup_n-D  BreakpointsForDimension1=ATQD_APSDecTimeGain_Y_s  BreakpointsForDimension2=ATQD_APSDecTimeGain_X_Deg  Table=MTQD_ForceAPSDecTimeGain_Z_c  InternalRulePriority=Speed  RndMeth=Simplest  InputSameDT=on
      settings: InputPortMap=u0,u1
  MTQD_PedPressDecTimeGain_Z_c : Lookup_n-D  BreakpointsForDimension1=ATQD_APSDecTimeGain_Y_s  BreakpointsForDimension2=ATQD_APSDecTimeGain_X_Deg  Table=MTQD_PedPressDecTimeGain_Z_c  InternalRulePriority=Speed  RndMeth=Simplest  InputSameDT=on
      settings: InputPortMap=u0,u1
  Max : MinMax  Function=max  Inputs=2
  NOT{1..3,5} (4 alike) : Logic  Operator=NOT  AllPortsSameDT=off  OutDataTypeStr=boolean
  OR : Logic  Operator=OR  AllPortsSameDT=off  OutDataTypeStr=boolean
  Product{,1..4} (5 alike) : Product
  Relational Operator : RelationalOperator  OutDataTypeStr=boolean  RndMeth=Simplest
  SR_Latch : hcu_lib/Basic_Blocks/SR_Latch
  Saturation Dynamic : simulink/Discontinuities/Saturation Dynamic  OutMin=[]  OutMax=[]  OutDataTypeStr=Inherit: Same as second input  OutDataType=fixdt(1, 16)  OutScaling=2^-10  DoSatur=off
  Switch{,1..4,9} (6 alike) : Switch  Criteria=u2 ~= 0
      settings: AttributesFormatString=%<Criteria>
  VTQD_APSDecReq_mps2 : Outport
  wires:
  [VTQD_APSDecReqTs_c] -> FirstOrderFilter1/3
  [VTQD_ActAPSPosn_pct] -> MTQD_APSDecReqTs_Y_c/1
  MTQD_APSDecReqTs_Y_c/1 -> [VTQD_APSDecReqTs_c]  "VTQD_APSDecReqTs_c"
  VTQD_ActAPSPosn_pct/1 -> [VTQD_ActAPSPosn_pct]
  task_time_s/1 -> [task_time_s]
  [task_time_s] -> FirstOrderFilter1/2
  FirstOrderFilter1/1 -> Switch1/3
  [VTQD_AutiHoldRelease_flg] -> NOT1/1
  Constant2/1 -> NOT3/1
  [VTQD_APSDecReqA_flg] -> AND1/1
  Switch1/1 -> [VTQD_APSDecReq_mps2]  "VTQD_APSDecReq_mps2"
  Switch3/1 -> Switch1/1, FirstOrderFilter1/1
  AND1/1 -> Switch1/2
  NOT3/1 -> AND1/2
  NOT1/1 -> AND1/3
  [VTQD_AutiHoldRelease_flg] -> NOT2/1
  NOT2/1 -> AND4/3
  AND4/1 -> Switch3/2
  SR_Latch/1 -> OR/2
  OR/1 -> Switch9/2  "VTQD_APSDecReqMax_flg"
  VTQD_AutiHoldRelease_flg/1 -> [VTQD_AutiHoldRelease_flg]
  [VTQD_AutiHoldRelease_flg] -> SR_Latch/2
  Switch9/1 -> Switch3/1
  [VTQD_APSReqTimer_s] -> Relational Operator/1
  Constant1/1 -> Relational Operator/2
  Relational Operator/1 -> SR_Latch/1
  Constant43/1 -> OR/1
  [VTQD_APSDecReq_mps2] -> VTQD_APSDecReq_mps2/1
  VTQD_APSDecReqA_flg/1 -> [VTQD_APSDecReqA_flg]
  VVMC_EstSlope_Deg/1 -> [VVMC_EstSlope_Deg]
  VTQD_APSReqTimer_s/1 -> [VTQD_APSReqTimer_s]
  VVMC_LongAcc_Gps/1 -> [VVMC_LongAcc_Gps]
  VTQD_VehActSpd_kph/1 -> [VTQD_VehActSpd_kph]
  Constant8/1 -> Product1/2
  Constant22/1 -> Saturation Dynamic/3
  [VTQD_APSDecReqCMD_mps2] -> Add/1
  NOT5/1 -> AND4/2
  [VTQD_APSDecReqA_flg] -> AND4/1
  [VTQD_VehActSpd_kph] -> MTQD_APSDecReqCMD_Y_mps2/1
  Product1/1 -> Add/2
  [VTQD_APSReqTimer_s] -> MTQD_APSDecTimeGain_Z_c/1
  [VTQD_VehActSpd_kph] -> MTQD_APSDecReg_Z_mps2/2
  Add/1 -> Saturation Dynamic/2
  Constant19/1 -> NOT5/1
  [VTQD_MapAPSDecReg_mps2] -> Product2/1
  [VVMC_LongAcc_Gps] -> Product1/1
  MTQD_APSDecReqCMD_Y_mps2/1 -> [VTQD_APSDecReqCMD_mps2]  "VTQD_APSDecReqCMD_mps2"
  Constant13/1 -> Switch3/3
  MTQD_APSDecReg_Z_mps2/1 -> [VTQD_MapAPSDecReg_mps2]  "VTQD_MapAPSDecReq_mps2"
  Constant21/1 -> Saturation Dynamic/1
  [VTQD_APSDecTimeGain_c] -> Product2/2
  [VVMC_EstSlope_Deg] -> MTQD_APSDecTimeGain_Z_c/2
  Saturation Dynamic/1 -> MTQD_APSDecReg_Z_mps2/1, [VTQD_ActOPDHoldAccDev_mps2]  "VTQD_ActOPDHoldAccDev_mps2"
  [VTQD_ActOPDHoldAccDev_mps2] -> MTQD_ForceAPSDecReq_Z_mps2/1
  MTQD_ForceAPSDecReq_Z_mps2/1 -> [VTQD_ForceMapAPSDecReq_mps2]  "VTQD_ForceMapAPSDecReq_mps2"
  [VTQD_VehActSpd_kph] -> MTQD_ForceAPSDecReq_Z_mps2/2
  [VTQD_LowIdleAccPedal_flg] -> Switch4/2
  MTQD_PedPressDecTimeGain_Z_c/1 -> Switch4/1  "VTQD_PedPressDecTimeGain_c"
  [VVMC_EstSlope_Deg] -> MTQD_PedPressDecTimeGain_Z_c/2
  [VTQD_APSReqTimer_s] -> MTQD_PedPressDecTimeGain_Z_c/1
  Switch4/1 -> [VTQD_APSDecTimeGain_c]  "VTQD_APSDecTimeGain_c"
  MTQD_APSDecTimeGain_Z_c/1 -> Switch4/3
  MTQD_ForceAPSDecTimeGain_Z_c/1 -> [VTQD_ForceAPSDecTimeGain_c]  "VTQD_ForceAPSDecTimeGain_c"
  [VVMC_EstSlope_Deg] -> MTQD_ForceAPSDecTimeGain_Z_c/2
  [VTQD_APSReqTimer_s] -> MTQD_ForceAPSDecTimeGain_Z_c/1
  [VTQD_APSDecTimeGain_c] -> Product/2
  [VTQD_APSDecReq_mps2] -> Delay/1
  Product/1 -> Switch/3
  [VTQD_ForceMapAPSDecReq_mps2] -> Product3/1
  [VTQD_ForceAPSDecTimeGain_c] -> Product3/2
  Max/1 -> Switch9/1
  Product3/1 -> Switch/1
  Delay/1 -> Max/2
  Switch/1 -> Max/1
  [VTQD_OPDHoldForceEn_flg] -> Switch/2
  [VTQD_MapAPSDecReg_mps2] -> Product/1
  [VTQD_ForceAPSDecTimeGain_c] -> Product4/2
  [VTQD_ForceMapAPSDecReq_mps2] -> Product4/1
  Product4/1 -> Switch2/1
  [VTQD_OPDHoldForceEn_flg] -> Switch2/2
  Switch2/1 -> Switch9/3
  Product2/1 -> Switch2/3
  VTQD_LowIdleAccPedal_flg/1 -> [VTQD_LowIdleAccPedal_flg]
  VTQD_OPDHoldForceEn_flg/1 -> [VTQD_OPDHoldForceEn_flg]
